simulink model "motores"  (R2015b)
settings: Solver=VariableStepAuto  StartTime=0.0  StopTime=10.0  RelTol=1e-3
values from neighbouring files (symbols this model uses):
  Den_Derecha = [(Inercia_Total*L_Derecha) (Ra_Derecha*Inercia_Total+L_Derecha*Bm_Derecha) (Ra_Derecha*Bm_Derecha+Kv_Derecha*Kv_Derecha)]    [Motor_DC.m]    (also in Motores.mat = [5.234727e-09 3.9497430885e-05 0.080724317205])
  Den_Izquierda = [(Inercia_Total*L_Izquierda) (Ra_Izquierda*Inercia_Total+L_Izquierda*Bm_Izquierda) (Ra_Izquierda*Bm_Izquierda+Kv_Izquierda*Kv_Izquierda)]    [Motor_DC.m]    (also in Motores.mat = [5.108589e-09 4.1835350431e-05 0.105046154423])
  Num_Derecha = Kv_Derecha    (= 0.2121)    [Motor_DC.m]    (also in Motores.mat)
  Num_Izquierda = Kv_Izquierda    (= 0.2304)    [Motor_DC.m]    (also in Motores.mat)
settings Model: Creator=Anna Cafaro  LastModifiedBy=Anna Cafaro

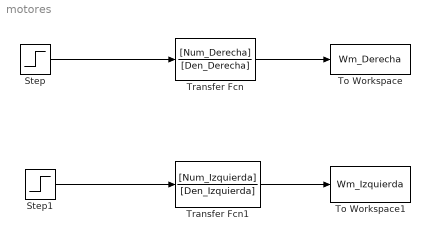
== system motores ==
  Step : Step  After=0.529
  Step1 : Step  After=0.5
  To Workspace : ToWorkspace  VariableName=Wm_Derecha  SampleTime=-1
  To Workspace1 : ToWorkspace  VariableName=Wm_Izquierda  SampleTime=-1
  "Transfer Fcn " : TransferFcn  Numerator=[Num_Derecha]  Denominator=[Den_Derecha]
  Transfer Fcn1 : TransferFcn  Numerator=[Num_Izquierda]  Denominator=[Den_Izquierda]
  wires:
  Step/1 -> "Transfer Fcn "/1
  "Transfer Fcn "/1 -> To Workspace/1
  Step1/1 -> Transfer Fcn1/1
  Transfer Fcn1/1 -> To Workspace1/1
